simulink model "group1_control_submission"  (R2024a)
settings: Solver=VariableStepAuto  StartTime=0.0  StopTime=10.0  RelTol=1e-3
settings Model: Creator=Riley  LastModifiedBy=Riley

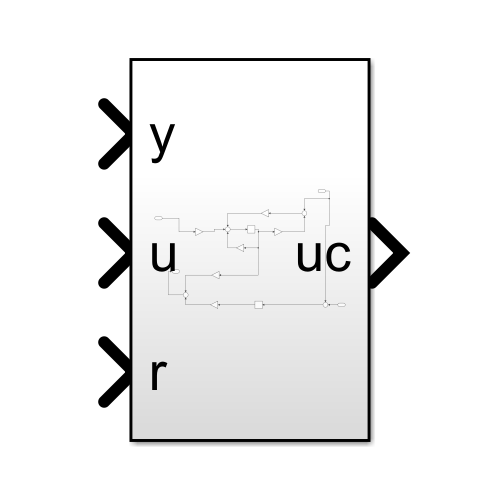
[thumbnail: Simulink's stored preview of the top-level diagram]
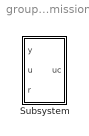
== system group1_control_submission ==
  Subsystem : Subsystem

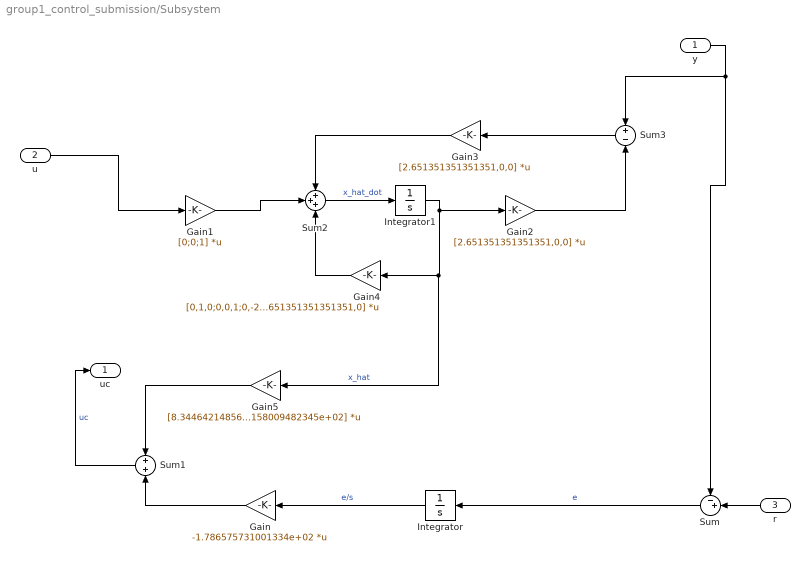
== system group1_control_submission/Subsystem ==
  y : Inport
  u : Inport  Port=2
  r : Inport  Port=3
  Gain : Gain  Gain=-1.786575731001334e+02  Multiplication=Matrix(K*u)
  Gain1 : Gain  Gain=[0;0;1]  Multiplication=Matrix(K*u)
  Gain2 : Gain  Gain=[2.651351351351351,0,0]  Multiplication=Matrix(K*u)
  Gain3 : Gain  Gain=[2.651351351351351,0,0]  Multiplication=Matrix(K*u)
  Gain4 : Gain  Gain=[0,1,0;0,0,1;0,-2.651351351351351,0]  Multiplication=Matrix(K*u)
  Gain5 : Gain  Gain=[8.344642148564543e+02,3.081129663116928e+02,1.833158009482345e+02]  Multiplication=Matrix(K*u)
  Integrator : Integrator
  Integrator1 : Integrator
  Sum : Sum  Inputs=-+|
  Sum1 : Sum  Inputs=+|+
  Sum2 : Sum  Inputs=+++
  Sum3 : Sum  Inputs=+|-
  uc : Outport
  wires:
  Gain/1 -> Sum1/2
  Integrator1/1 -> Gain5/1, Gain4/1, Gain2/1  "x_hat"
  Sum/1 -> Integrator/1  "e"
  y/1 -> Sum3/1, Sum/1
  Sum2/1 -> Integrator1/1  "x_hat_dot"
  Sum1/1 -> uc/1  "uc"
  Gain4/1 -> Sum2/3
  Gain2/1 -> Sum3/2
  Gain3/1 -> Sum2/1
  Gain5/1 -> Sum1/1
  Gain1/1 -> Sum2/2
  Sum3/1 -> Gain3/1
  Integrator/1 -> Gain/1  "e/s"
  u/1 -> Gain1/1
  r/1 -> Sum/2
